simulink model "CyclingProcess"  (R2022a)
settings: configuration reference "MainConfig" (kept outside this file)
PostLoadFcn:
  | load('input_modelo_bateria.mat')
undefined symbols (not defined in the file or in its folder): rest_time, SOC_MAX, SOC_MIN, Temperature
libraries: fl_lib x1, nesl_utility x1
settings Model: PacingRate=1000  Creator=eduardo.guimaraes  LastModifiedBy=mateu
settings ConfigSetRef: SourceName=MainConfig  SourceLocation=Base Workspace

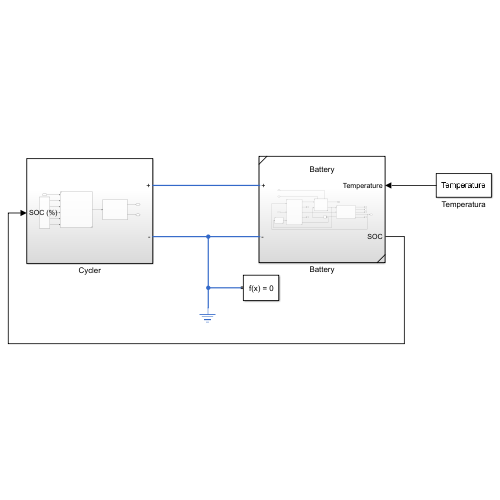
[thumbnail: Simulink's stored preview of the top-level diagram]
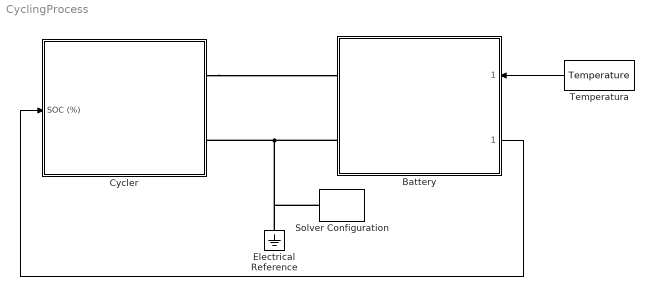
== system CyclingProcess ==
  Battery : Subsystem  ReferencedSubsystem=Battery
      settings: PortSchema="{\"entries\":[{\"content\":{\"sides\":[{\"content\":{\"connectorIds\":[\"LConn1\",\"LConn2\"]},\"type\":\"ConnectorPlacement.EquallySpacedRectSide\",\"uuid\":\"a87e55b6-8336-4e26-8f41-032772011576\"},{\"content\":{\"connectorIds\":[\"In1\",\"Out1\"],\"side\":\"RIGHT\"},\"type\":\"ConnectorPlacement.EquallySpacedRectSide\",\"uuid\":\"bc789b5a-3568-4714-b987-1664b39aeefc\"},{\"content\":{\"connectorIds\":[],\"side\":\"TOP\"},\"type\":\"ConnectorPlacement.EquallySpacedRectSide\",\"uuid\":\"55da7c3a-53ce-47ce-bfe0-b863d0f3c76f\"}]},\"type\":\"ConnectorPlacement.EquallySpacedConnector\",\"uuid\":\"55ad2f4b-f4c7-4c3b-9b32-7be0611d2703\"}],\"packageUris\":[\"http://schema.mathworks.com/mf0/Connector/R2020b\"],\"version\":\"1.0\"}"
  Cycler : Subsystem
  Electrical Reference : fl_lib/Electrical/Electrical Elements/Electrical Reference
      settings: SourceProductBaseCode=PW,SS,VE
  Solver Configuration : nesl_utility/Solver Configuration  PhysicalDomain=network_engine_domain  SubClassName=solver  LeftPortType=input  RightPortType=generic  Tones=[]  Harmonics=[]  SimulateNoise=off  Profile=off  UseLocalSampling=off  EnableSwitchedLinearOptims=on  FrequencyDomain=off  UseCCode=off  RelTol=0.001  AbsTol=0.001  MinStep=1e-09  ToWorkspace=off  RevertToSquareIcSolve=off  NumHomotopyIterations=100  PhasorMode=off  PhasorModeNumHarmonics=1  IndexReductionMethod=DerivativeReplacement  DoDC=off  ResidualTolerance=1e-03  UseLocalSolver=off  LocalSolverChoice=NE_BACKWARD_EULER_ADVANCER  LocalSolverSampleTime=0.001  DoFixedCost=off  MaxNonlinIter=3  MaxModeIter=2  ComputeImpulses=off  ImpulseIterations=2  LinearAlgebra=auto  LinearAlgebraNumThread=0  EquationFormulation=NE_TIME_EF  DelaysMemoryBudget=1024  AutomaticFiltering=off  FilteringTimeConstant=0.001  PartitionStorageMethod=AS_NEEDED  PartitionMemoryBudget=1024  PartitionMethod=ROBUST
      settings: SourceProductBaseCode=SS,PW,VE
  Temperatura : Constant  Value=Temperature
  wires:
  Battery/1 -> Cycler/1(SOC (%))
  Temperatura/1 -> Battery/1
  connections:
  Solver Configuration/RConn1 -- Electrical Reference/LConn1 -- Battery/LConn2 -- Cycler/RConn2
  Cycler/RConn1 -- Battery/LConn1

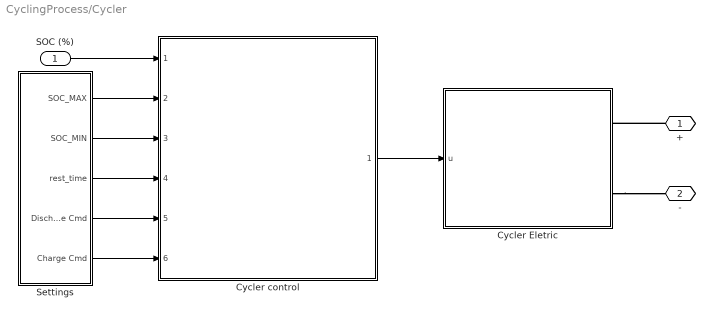
== system CyclingProcess/Cycler ==
  SOC (%) : Inport
  Cycler Eletric : Subsystem  Variant=on  VariantControl=Choice
  Cycler control : Subsystem  ReferencedSubsystem=cycling_control
  Settings : Subsystem  Variant=on  VariantControl=Choice
  + : PMIOPort  Side=Right
  - : PMIOPort  Port=2  Side=Right
  wires:
  SOC (%)/1 -> Cycler control/1
  Settings/1(SOC_MAX) -> Cycler control/2
  Settings/2(SOC_MIN) -> Cycler control/3
  Settings/3(rest_time) -> Cycler control/4
  Settings/4(Discharge Cmd) -> Cycler control/5
  Settings/5(Charge Cmd) -> Cycler control/6
  Cycler control/1 -> Cycler Eletric/1("u ")
  connections:
  Cycler Eletric/RConn2 -- -/RConn1
  +/RConn1 -- Cycler Eletric/RConn1

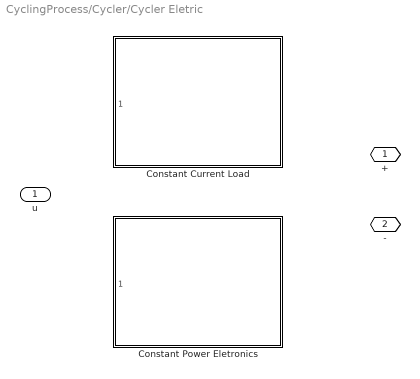
== system CyclingProcess/Cycler/Cycler Eletric ==
  "u " : Inport
  Constant Current Load : Subsystem  VariantControl=CYCLING_MODE == 0;  ReferencedSubsystem=constant_current_load
  Constant Power Eletronics : Subsystem  VariantControl=CYCLING_MODE == 1;  ReferencedSubsystem=constant_power_eletronics
  + : PMIOPort  Side=Right
  - : PMIOPort  Port=2  Side=Right

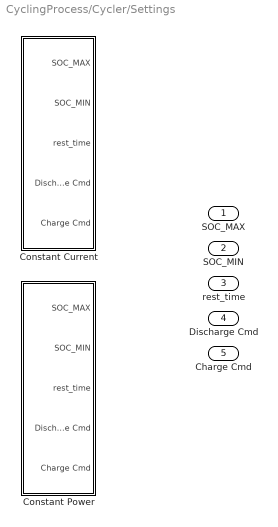
== system CyclingProcess/Cycler/Settings ==
  Constant Current : Subsystem  VariantControl=CYCLING_MODE == 0;
  Constant Power : Subsystem  VariantControl=CYCLING_MODE == 1;
  SOC_MAX : Outport
  SOC_MIN : Outport  Port=2
  rest_time : Outport  Port=3
  Discharge Cmd : Outport  Port=4
  Charge Cmd : Outport  Port=5

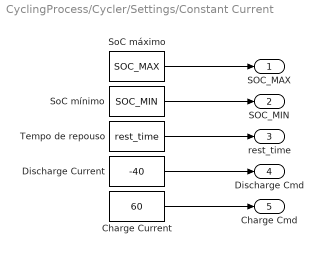
== system CyclingProcess/Cycler/Settings/Constant Current ==
  Charge Current : Constant  Value=60
  Discharge Current : Constant  Value=-40
  SoC máximo : Constant  Value=SOC_MAX
  SoC mínimo : Constant  Value=SOC_MIN
  Tempo de repouso : Constant  Value=rest_time
  SOC_MAX : Outport
  SOC_MIN : Outport  Port=2
  rest_time : Outport  Port=3
  Discharge Cmd : Outport  Port=4
  Charge Cmd : Outport  Port=5
  wires:
  SoC máximo/1 -> SOC_MAX/1
  Discharge Current/1 -> Discharge Cmd/1
  SoC mínimo/1 -> SOC_MIN/1
  Tempo de repouso/1 -> rest_time/1
  Charge Current/1 -> Charge Cmd/1

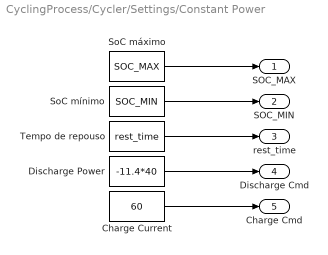
== system CyclingProcess/Cycler/Settings/Constant Power ==
  Charge Current : Constant  Value=60
  Discharge Power : Constant  Value=-11.4*40
  SoC máximo : Constant  Value=SOC_MAX
  SoC mínimo : Constant  Value=SOC_MIN
  Tempo de repouso : Constant  Value=rest_time
  SOC_MAX : Outport
  SOC_MIN : Outport  Port=2
  rest_time : Outport  Port=3
  Discharge Cmd : Outport  Port=4
  Charge Cmd : Outport  Port=5
  wires:
  SoC máximo/1 -> SOC_MAX/1
  Discharge Power/1 -> Discharge Cmd/1
  SoC mínimo/1 -> SOC_MIN/1
  Tempo de repouso/1 -> rest_time/1
  Charge Current/1 -> Charge Cmd/1
